simulink library "INT_InjCrv_PiIAddCor"  (R2016b)
settings: Solver=VariableStepAuto  StartTime=0.0  StopTime=10.0  RelTol=1e-3
settings Model: Creator=Administrator  LastModifiedBy=Administrator

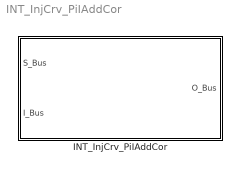
== system INT_InjCrv_PiIAddCor ==
  INT_InjCrv_PiIAddCor : Subsystem

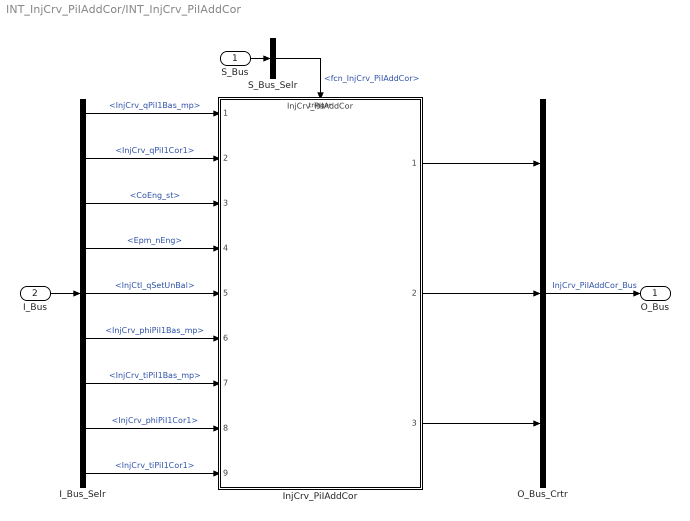
== system INT_InjCrv_PiIAddCor/INT_InjCrv_PiIAddCor ==
  S_Bus : Inport
  I_Bus : Inport  Port=2
  I_Bus_Selr : BusSelector  OutputSignals=InjCrv_qPiI1Bas_mp,InjCrv_qPiI1Cor1,CoEng_st,Epm_nEng,InjCtl_qSetUnBal,InjCrv_phiPiI1Bas_mp,InjCrv_tiPiI1Bas_mp,InjCrv_phiPiI1Cor1,InjCrv_tiPiI1Cor1
  InjCrv_PiIAddCor : ModelReference  ModelNameDialog=InjCrv_PiIAddCor  SimulationMode=Normal  ModelReferenceVersion=1.17  TriggerPortName=function  TriggerPortTriggerType=function-call  TriggerPortStatesWhenEnabling=held
  O_Bus_Crtr : BusCreator  Inputs=3
  S_Bus_Selr : BusSelector  OutputSignals=fcn_InjCrv_PiIAddCor
  O_Bus : Outport
  wires:
  S_Bus_Selr/1 -> InjCrv_PiIAddCor/Trigger  "<fcn_InjCrv_PiIAddCor>"
  S_Bus/1 -> S_Bus_Selr/1
  I_Bus/1 -> I_Bus_Selr/1
  I_Bus_Selr/1 -> InjCrv_PiIAddCor/1  "<InjCrv_qPiI1Bas_mp>"
  I_Bus_Selr/2 -> InjCrv_PiIAddCor/2  "<InjCrv_qPiI1Cor1>"
  I_Bus_Selr/3 -> InjCrv_PiIAddCor/3  "<CoEng_st>"
  I_Bus_Selr/4 -> InjCrv_PiIAddCor/4  "<Epm_nEng>"
  I_Bus_Selr/5 -> InjCrv_PiIAddCor/5  "<InjCtl_qSetUnBal>"
  I_Bus_Selr/6 -> InjCrv_PiIAddCor/6  "<InjCrv_phiPiI1Bas_mp>"
  I_Bus_Selr/7 -> InjCrv_PiIAddCor/7  "<InjCrv_tiPiI1Bas_mp>"
  I_Bus_Selr/8 -> InjCrv_PiIAddCor/8  "<InjCrv_phiPiI1Cor1>"
  I_Bus_Selr/9 -> InjCrv_PiIAddCor/9  "<InjCrv_tiPiI1Cor1>"
  O_Bus_Crtr/1 -> O_Bus/1  "InjCrv_PiIAddCor_Bus"
  InjCrv_PiIAddCor/1 -> O_Bus_Crtr/1
  InjCrv_PiIAddCor/2 -> O_Bus_Crtr/2
  InjCrv_PiIAddCor/3 -> O_Bus_Crtr/3
